simulink model "laufkatze_motor"  (R2020a)
settings: Solver=VariableStepAuto  StartTime=0.0  StopTime=10.0  RelTol=1e-3
settings Model: Creator=Andy  LastModifiedBy=Andy

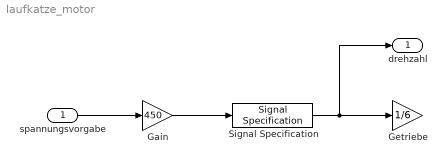
== system laufkatze_motor ==
  spannungsvorgabe : Inport  OutMin=[-10]  OutMax=[10]  Unit=1
  Gain : Gain  Gain=450
  Getriebe : Gain  Gain=1/6
  Signal Specification : SignalSpecification  Unit=1/min
  drehzahl : Outport  OutMin=[-4500]  OutMax=[4500]  Unit=1/min
  wires:
  Gain/1 -> Signal Specification/1
  spannungsvorgabe/1 -> Gain/1
  Signal Specification/1 -> Getriebe/1, drehzahl/1
